simulink model "unipolar"  (R2021a)
settings: Solver=VariableStepAuto  StartTime=0.0  StopTime=10.0  RelTol=1e-3
libraries: spsIGBTLib x4, simulink x3, spsSawtoothGeneratorLib x2, spsDCVoltageSourceLib x1, spsSeriesRLCBranchLib x1, spsVoltageMeasurementLib x1, spspowerguiLib x1
settings Model: Creator=furka  LastModifiedBy=furka

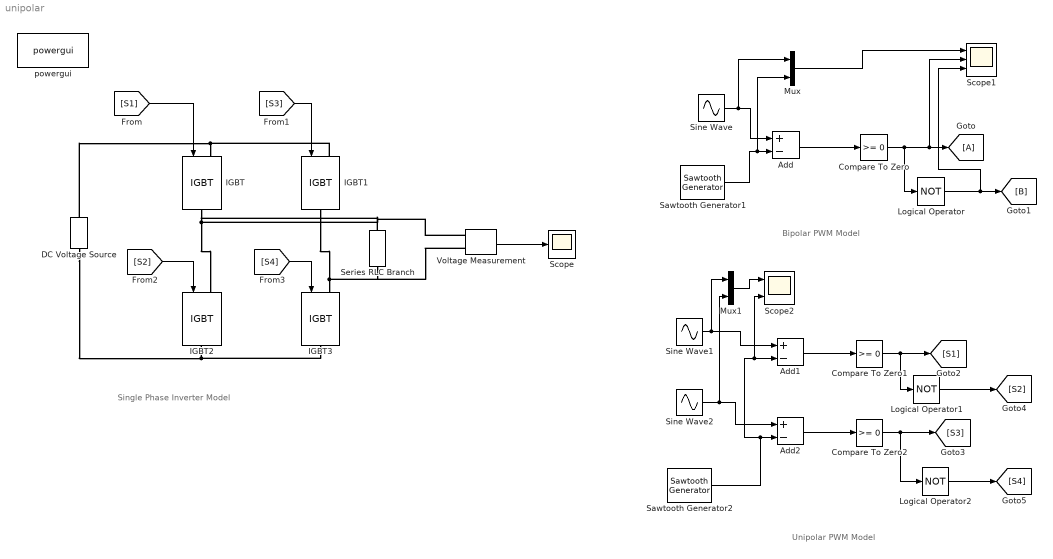
== system unipolar ==
  note: Unipolar PWM Model
  note: Bipolar PWM Model
  note: Single Phase Inverter Model
  Add : Sum  Inputs=+-
  Add1 : Sum  Inputs=+-
  Add2 : Sum  Inputs=+-
  Compare To Zero : simulink/Logic and Bit Operations/Compare To Zero  relop=>=  OutDataTypeStr=boolean
  Compare To Zero1 : simulink/Logic and Bit Operations/Compare To Zero  relop=>=  OutDataTypeStr=boolean
  Compare To Zero2 : simulink/Logic and Bit Operations/Compare To Zero  relop=>=  OutDataTypeStr=boolean
  DC Voltage Source : spsDCVoltageSourceLib/DC Voltage Source  Amplitude=100  Measurements=None
  IGBT{,1..3} (4 alike) : spsIGBTLib/IGBT  Ron=0.001  Lon=0  Vf=1  Tf=1e-6  Tt=2e-6  IC=0  Rs=1e5  Cs=inf  Measurements=off
  Logical Operator : Logic  Operator=NOT  AllPortsSameDT=off  OutDataTypeStr=boolean
  Logical Operator1 : Logic  Operator=NOT  Inputs=1  AllPortsSameDT=off  OutDataTypeStr=boolean
  Logical Operator2 : Logic  Operator=NOT  Inputs=1  AllPortsSameDT=off  OutDataTypeStr=boolean
  Mux : Mux  Inputs=2
  Mux1 : Mux  Inputs=2
  Sawtooth Generator1 : spsSawtoothGeneratorLib/Sawtooth Generator  Freq=1e3  Phase=180  Ts=0
  Sawtooth Generator2 : spsSawtoothGeneratorLib/Sawtooth Generator  Freq=1e3  Phase=180  Ts=0
  Scope : Scope
  Scope1 : Scope  NumInputPorts=3
  Scope2 : Scope  NumInputPorts=2
  Series RLC Branch : spsSeriesRLCBranchLib/Series RLC Branch  LConnTagsString=__new0  RConnTagsString=__new0  BranchType=R  Resistance=1  Inductance=1e-3  SetiL0=off  InitialCurrent=0  Capacitance=1e-6  Setx0=off  InitialVoltage=0  Measurements=None
  Sine Wave : Sin  Frequency=2*pi*50  SampleTime=0
  Sine Wave1 : Sin  Frequency=2*pi*50  SampleTime=0
  Sine Wave2 : Sin  Frequency=2*pi*50  Phase=pi  SampleTime=0
  Voltage Measurement : spsVoltageMeasurementLib/Voltage Measurement  PhasorSimulation=off  OutputType=Complex  PSBequivalent=0
  powergui : spspowerguiLib/powergui  Priority=1  SimulationMode=Continuous  SampleTime=50e-6  frequency=60  Iterations=50  frequencyindice=0  Pbase=100e6  ErrMax=1e-4  UnitsV=kV  UnitsW=MW  buscounter=0  FunctionMessages=off  echomessages=off  EnableUseOfTLC=off  CurrentSourceSwitches=off  DisableSnubberDevices=off  DisableRonSwitches=off  DisableVfSwitches=off  DisplayEquations=off  AutomaticDiscreteSolvers=off  SolverType=Tustin/Backward Euler (TBE)  Interpol=off  ExternalGateDelay=off  methode=off  Ts=100  x0status=blocks  SPID=on  SwTol=0  HookPort=off  NonlinearTolerance=1e-4  nMaxIteration=100  ContinueOnMaxIteration=off  RestoreLinks=warning  ResistiveCurrentMeasurement=off  Frange=[0:2:500]  Ylog=off  Xlog=on  ShowGrid=off  save=off  variable=ZData  structure=0  ZoomFFT=off  StartTime=0.0  cycles=1  DisplayStyle=1  fundamental=60  FreqAxis=off  MaxFrequency=1000  frequencyindicesteady=1  RmsSteady=1  display=off
  wires:
  [S2] -> IGBT2/1
  [S4] -> IGBT3/1
  [S3] -> IGBT1/1
  [S1] -> IGBT/1
  Voltage Measurement/1 -> Scope/1
  Sine Wave/1 -> Mux/1, Add/1
  Sawtooth Generator1/1 -> Mux/2, Add/2
  Add/1 -> Compare To Zero/1
  Compare To Zero/1 -> Logical Operator/1, Scope1/2, [A]
  Logical Operator/1 -> Scope1/3, [B]
  Mux/1 -> Scope1/1
  Sine Wave1/1 -> Mux1/1, Add1/1
  Sine Wave2/1 -> Mux1/2, Add2/1
  Sawtooth Generator2/1 -> Scope2/2, Add1/2, Add2/2
  Add1/1 -> Compare To Zero1/1
  Add2/1 -> Compare To Zero2/1
  Compare To Zero2/1 -> Logical Operator2/1, [S3]
  Compare To Zero1/1 -> Logical Operator1/1, [S1]
  Logical Operator1/1 -> [S2]
  Logical Operator2/1 -> [S4]
  Mux1/1 -> Scope2/1
  connections:
  DC Voltage Source/RConn1 -- IGBT1/LConn1 -- IGBT/LConn1
  DC Voltage Source/LConn1 -- IGBT3/RConn1 -- IGBT2/RConn1
  IGBT1/RConn1 -- Voltage Measurement/LConn2 -- Series RLC Branch/RConn1 -- IGBT3/LConn1
  IGBT/RConn1 -- Voltage Measurement/LConn1 -- Series RLC Branch/LConn1 -- IGBT2/LConn1
